simulink model "fromiWalker"  (R2014a)
settings: Solver=ode45  StartTime=0.0  StopTime=Inf  RelTol=1e-3
InitFcn:
  | Ts=0.01
  | lid = LIDAR();
  | rob = DifferentialRobot();
  | rob.dt = Ts;
  | rob.attachLidar(lid, [0.6,0,0]);
  | close all;
  | figure;
  | axis equal;
  | hold on;
  | whitebg([0 0 0]);
  | grid on;
  | axis([-10 10 -10 10]);
  | pl = Plotter(gca);
libraries: iWalkerLib x3
settings Model: Creator=Brian  LastModifiedBy=Brian

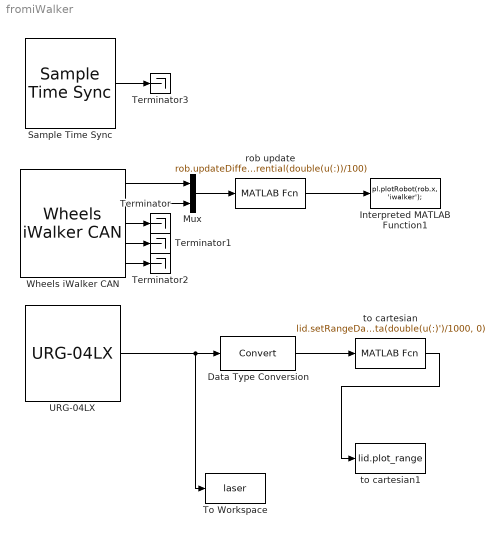
== system fromiWalker ==
  Data Type Conversion : DataTypeConversion
  Interpreted MATLAB Function1 : MATLABFcn  MATLABFcn=pl.plotRobot(rob.x, 'iwalker');  OutputDimensions=0
  Mux : Mux  Inputs=2
  Sample Time Sync : iWalkerLib/Sample Time Sync  Priority=8
  Terminator{,1..3} (4 alike) : Terminator
  To Workspace : ToWorkspace  VariableName=laser  SaveFormat=Structure With Time  SampleTime=-1
  URG-04LX : iWalkerLib/URG-04LX  COM=1  SampleTime=0.5  Verbose=off
  Wheels iWalker CAN : iWalkerLib/Wheels iWalker CAN  SystemSampleTime=-1
  rob update : MATLABFcn  MATLABFcn=rob.updateDifferential(double(u(:))/100)
  to cartesian : MATLABFcn  MATLABFcn=lid.setRangeData(double(u(:)')/1000, 0)
  to cartesian1 : MATLABFcn  MATLABFcn=lid.plot_range  OutputDimensions=0  Output1D=off
  wires:
  Wheels iWalker CAN/1 -> Mux/1
  Wheels iWalker CAN/2 -> Mux/2
  Wheels iWalker CAN/3 -> Terminator/1
  Wheels iWalker CAN/4 -> Terminator1/1
  Wheels iWalker CAN/5 -> Terminator2/1
  Sample Time Sync/1 -> Terminator3/1
  Mux/1 -> rob update/1
  rob update/1 -> Interpreted MATLAB Function1/1
  Data Type Conversion/1 -> to cartesian/1
  URG-04LX/1 -> To Workspace/1, Data Type Conversion/1
  to cartesian/1 -> to cartesian1/1
